simulink model "lc_2_step_strategy"  (R2019a)
settings: Solver=VariableStepAuto  StartTime=0.0  StopTime=15  RelTol=1e-3
values from neighbouring files (symbols this model uses):
  a1 = 2*(Cf+Cr)/vehMass    [SimulinkScenario.m]
  a2 = 2*(Cf*lf-Cr*lr)/vehMass    [SimulinkScenario.m]
  b1 = 2*Cf/vehMass    [SimulinkScenario.m]
  maxDelta = 25*pi/180    (= 0.436332312999)    [sim_parameters.m]
  maxDeltaDot = 9.4*pi/180    (= 0.164060949687)    [sim_parameters.m]
  maxLatJerk = 0.67    [sim_parameters.m]
libraries: autolibshared x1, simulink x1
settings Model: Creator=Fernando VM  LastModifiedBy=Fernando VM

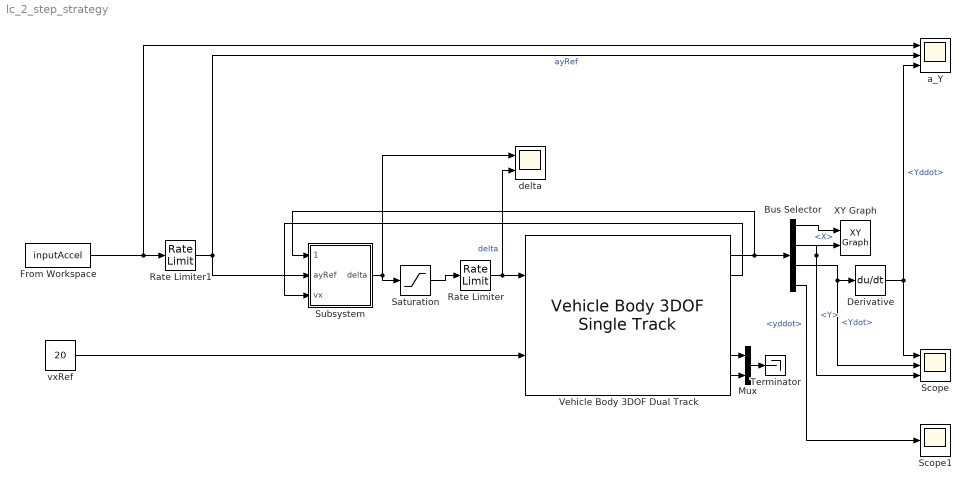
== system lc_2_step_strategy ==
  Bus Selector : BusSelector  OutputSignals=InertFrm.Cg.Disp.X,InertFrm.Cg.Disp.Y,InertFrm.Cg.Vel.Ydot,BdyFrm.Cg.Acc.yddot
  Derivative : Derivative
  From Workspace : FromWorkspace  VariableName=inputAccel  SampleTime=0
  Mux : Mux  Inputs=2
  Rate Limiter : RateLimiter  RisingSlewLimit=maxDeltaDot  FallingSlewLimit=-maxDeltaDot  SampleTimeMode=inherited
  Rate Limiter1 : RateLimiter  RisingSlewLimit=maxLatJerk  FallingSlewLimit=-maxLatJerk  SampleTimeMode=inherited
  Saturation : Saturate  UpperLimit=maxDelta  LowerLimit=-maxDelta
  Scope : Scope  NumInputPorts=3
  Scope1 : Scope
  Subsystem : Subsystem
  Terminator : Terminator
  Vehicle Body 3DOF Dual Track : autolibshared/Vehicle Body 3DOF Single Track  trackMode=Single (bicycle)  inputMode=External longitudinal velocity  frontSteerMode=on  rearSteerMode=off  windMode=off  muMode=off  extFMode=off  extMMode=off  extXo=off  extpsio=off  extxdoto=off  extro=off  extYo=off  extTamb=off  extydoto=off  aMode=2  NF=2  NR=2  m=2000  a=1.4  b=1.6  h=0.35  X_o=0  xdot_o=0  CalphaMode=off  sigmaMode=on  d=0  w=[1.4,1.4]  Cy_f=12e3  Cy_r=11e3  sigma_f=.1  sigma_r=.1  alpha_f_brk=[-.1 .1]  Cy_f_data=[-9e3 9e3]  alpha_r_brk=[-.1 .1]  Cy_r_data=[-9e3 9e3]  Y_o=0  ydot_o=0  Izz=4000  psi_o=0  r_o=0  Af=2  Cd=.3  Cl=.1  Cpm=.1  beta_w=[0:0.01:0.3]  Cs=[0:0.03:0.9]  Cym=[0:0.01:0.3]  Pabs=101325  Tair=273  g=9.81  mu=1  xdot_tol=.01  Fznom=5000  Fxtire_sat=7e4  Fytire_sat=7e4  longOff=0  latOff=0  vertOff=0  wrapAng=off
      settings: SourceProductName=Powertrain Blockset  SourceProductBaseCode=PW
  XY Graph : simulink/Sinks/XY Graph  xmin=-1  xmax=250  ymin=-1  ymax=10  st=-1
  a_Y : Scope  NumInputPorts=3
  delta : Scope  NumInputPorts=2
  vxRef : Constant  Value=20
  wires:
  Saturation/1 -> Rate Limiter/1
  Rate Limiter/1 -> delta/2, Vehicle Body 3DOF Dual Track/1  "delta"
  From Workspace/1 -> a_Y/1, Rate Limiter1/1
  Rate Limiter1/1 -> Subsystem/2(ayRef), a_Y/2  "ayRef"
  Vehicle Body 3DOF Dual Track/1 -> Bus Selector/1, Subsystem/1(states)
  vxRef/1 -> Vehicle Body 3DOF Dual Track/2
  Subsystem/1(delta) -> delta/1, Saturation/1
  Vehicle Body 3DOF Dual Track/6 -> Mux/1
  Vehicle Body 3DOF Dual Track/7 -> Mux/2
  Vehicle Body 3DOF Dual Track/2 -> Subsystem/3(vx)
  Mux/1 -> Terminator/1
  Bus Selector/1 -> XY Graph/1  "<X>"
  Bus Selector/2 -> Scope/3, XY Graph/2  "<Y>"
  Bus Selector/3 -> Scope/2, Derivative/1  "<Ydot>"
  Derivative/1 -> Scope/1, a_Y/3  "<Yddot>"
  Bus Selector/4 -> Scope1/1  "<yddot>"

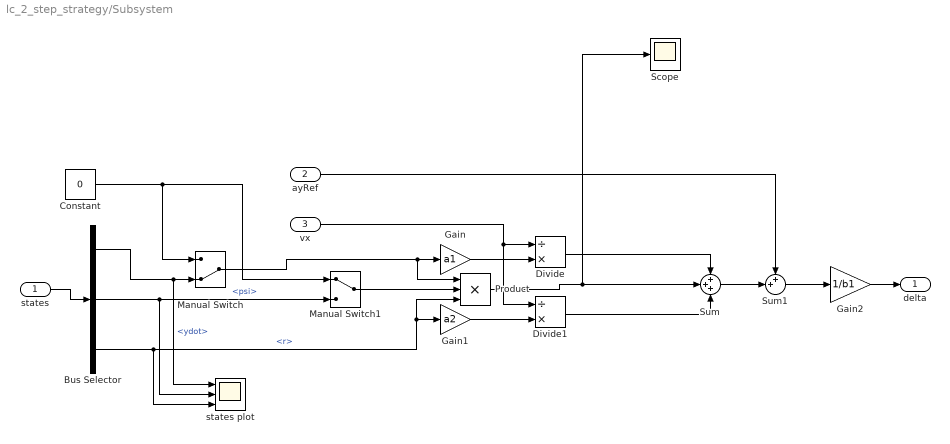
== system lc_2_step_strategy/Subsystem ==
  states : Inport
  ayRef : Inport  Port=2
  vx : Inport  Port=3
  Bus Selector : BusSelector  OutputSignals=BdyFrm.Cg.Vel.ydot,InertFrm.Cg.Ang.psi,BdyFrm.Cg.AngVel.r
  Constant : Constant  Value=0
  Divide : Product  Inputs=/*
  Divide1 : Product  Inputs=/*
  Gain : Gain  Gain=a1
  Gain1 : Gain  Gain=a2
  Gain2 : Gain  Gain=1/b1
  Manual Switch : ManualSwitch  CurrentSetting=0
  Manual Switch1 : ManualSwitch
  Product : Product  Inputs=***
  Scope : Scope
  Sum : Sum  Inputs=+++
  Sum1 : Sum  Inputs=++|
  states plot : Scope  NumInputPorts=3
  delta : Outport
  wires:
  states/1 -> Bus Selector/1
  Bus Selector/3 -> states plot/3, Product/3, Gain1/1  "<r>"
  Gain/1 -> Divide/2
  vx/1 -> Divide1/1, Divide/1
  Divide/1 -> Sum/1
  Divide1/1 -> Sum/3
  Sum/1 -> Sum1/2
  Sum1/1 -> Gain2/1
  ayRef/1 -> Sum1/1
  Gain1/1 -> Divide1/2
  Gain2/1 -> delta/1
  Constant/1 -> Manual Switch1/1, Manual Switch/1
  Product/1 -> Sum/2, Scope/1
  Manual Switch/1 -> Product/1, Gain/1
  Bus Selector/1 -> states plot/1, Manual Switch/2  "<ydot>"
  Manual Switch1/1 -> Product/2
  Bus Selector/2 -> states plot/2, Manual Switch1/2  "<psi>"
